simulink model "RL1"  (R2023a)
settings: Solver=FixedStepAuto  StartTime=0.0  StopTime=100  FixedStep=0.05  RelTol=1e-3  EnableMultiTasking=on
values from neighbouring files (symbols this model uses):
  Inz = 1538    [MAIN.m]
  Kx = zeros(n+1, n+1)    [MAIN.m]
  Kz = [K(2)      -K(2)    0         0         0         0    0 ... (first row only)    [MAIN.m]
  Mx = Mx + triu(Mx, 1)'    [MAIN.m]
  Mz = zeros(7,7)    [MAIN.m]
libraries: simulink x6, rllib x1
settings Model: ExtModeTrigDuration=10000  Creator=AUSIM-ZJD  LastModifiedBy=AUSIM-ZJD
settings SolverCC: AlgebraicLoopSolver=TrustRegion  PositivePriorityOrder=on
settings DataIOCC: ReturnWorkspaceOutputs=off
settings OptimizationCC: LifeSpan=inf
settings DebuggingCC: UnconnectedInputMsg=warning  UnconnectedOutputMsg=warning  UnconnectedLineMsg=warning  ArithmeticOperatorsInVariantConditions=warning
settings ModelReferenceCC: EnableRefExpFcnMdlSchedulingChecks=on
settings SFSimCC: SimUseLocalCustomCode=off  CustomCodeUndefinedFunction=UseInterfaceOnly
settings RTWCC: Description=QUARC Win64 Target  SystemTargetFile=quarc_win64.tlc  TemplateMakefile=quarc_default_tmf  RTWUseLocalCustomCode=off
settings CodeAppCC: StateflowObjectComments=on
settings STFCustomTargetCC: TargetPreCompLibLocation=C:\PROGRA~3\QUARC\lib\2016a\win64\release  UseToolchainInfoCompliant=off  SystemTargetFile=quarc_win64.tlc
settings GRTTargetCC: TargetPreCompLibLocation=C:\PROGRA~3\QUARC\lib\2016a\win64\release  ParMdlRefBuildCompliant=off  CompOptLevelCompliant=off  CombineOutputUpdateFcns=off  MatFileLogging=off  CPPClassGenCompliant=off  GRTInterface=on  UseToolchainInfoCompliant=off  ExtMode=on  ExtModeMexFile=quarc_comm
settings ConfigComp: CovMetricSettings=dswe

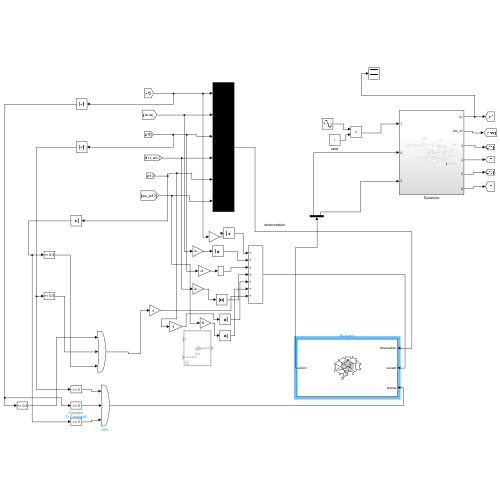
[thumbnail: Simulink's stored preview of the top-level diagram]
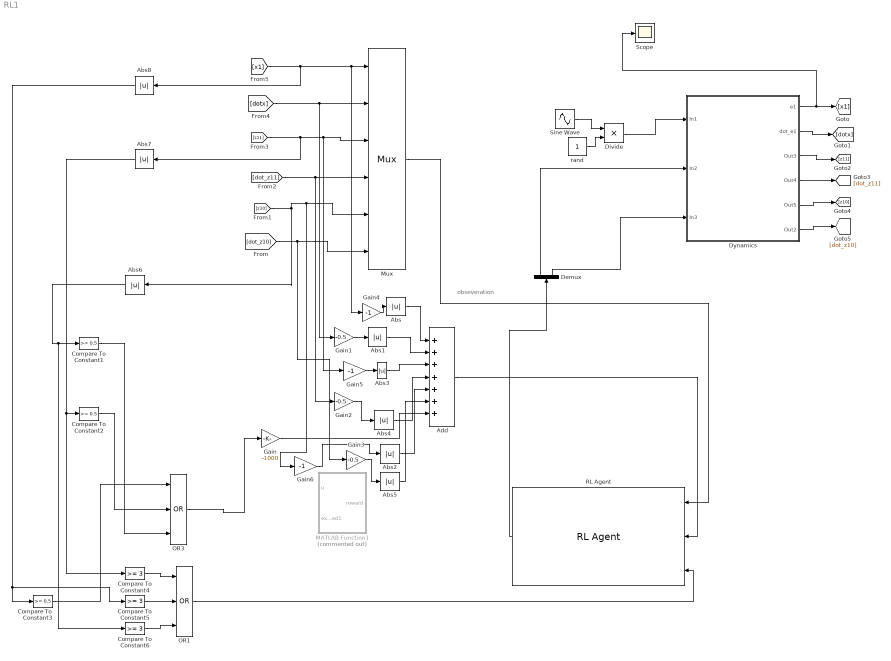
== system RL1 ==
  note: obseveration
  Abs{,1..8} (9 alike) : Abs  SaturateOnIntegerOverflow=off
  Add : Sum  Inputs=+++++++
  Compare To Constant1 : simulink/Logic and Bit Operations/Compare To Constant  relop=>=  const=0.5  OutDataTypeStr=boolean
  Compare To Constant2 : simulink/Logic and Bit Operations/Compare To Constant  relop=>=  const=0.5  OutDataTypeStr=boolean
  Compare To Constant3 : simulink/Logic and Bit Operations/Compare To Constant  relop=>=  const=0.5  OutDataTypeStr=boolean
  Compare To Constant4 : simulink/Logic and Bit Operations/Compare To Constant  relop=>=  const=3  OutDataTypeStr=boolean
  Compare To Constant5 : simulink/Logic and Bit Operations/Compare To Constant  relop=>=  const=3  OutDataTypeStr=boolean
  Compare To Constant6 : simulink/Logic and Bit Operations/Compare To Constant  relop=>=  const=3  OutDataTypeStr=boolean
  Demux : Demux  Outputs=2
  Divide : Product  Inputs=**
  Dynamics : Subsystem
  Gain : Gain  Gain=-1000
  Gain1 : Gain  Gain=-0.5
  Gain2 : Gain  Gain=-0.5
  Gain3 : Gain  Gain=-0.5
  Gain4 : Gain  Gain=-1
  Gain5 : Gain  Gain=-1
  Gain6 : Gain  Gain=-1
  MATLAB Function1 : MATLAB Function  Commented=on  TreatAsAtomicUnit=on
  Mux : Mux  Inputs=6
  OR1 : Logic  Operator=OR  Inputs=3  IconShape=distinctive  AllPortsSameDT=off  OutDataTypeStr=boolean
  OR3 : Logic  Operator=OR  Inputs=3  IconShape=distinctive  AllPortsSameDT=off  OutDataTypeStr=boolean
  RL Agent : rllib/RL Agent  Agent=agent  ExternalActionAsInput=off  ProvideLastAction=off  ProvideCumRwd=off  TreatAsDirectFeedthrough=on  UseStrictObservationDataTypes=off
  Scope : Scope
  Sine Wave : Sin  Amplitude=5000  SampleTime=0.05
  rand : Constant
  wires:
  Sine Wave/1 -> Divide/1
  Demux/2 -> Dynamics/3(In3)
  Dynamics/2(dot_e1) -> [dotx]
  Dynamics/6(Out2) -> [dot_z10]
  Dynamics/1(e1) -> Scope/1, [x1]
  Dynamics/3(Out3) -> [z11]
  Dynamics/4(Out4) -> [dot_z11]
  Dynamics/5(Out5) -> [z10]
  [dotx] -> Mux/2, Gain1/1
  [dot_z10] -> Gain3/1, Mux/6
  Mux/1 -> RL Agent/1
  [dot_z11] -> Gain2/1, Mux/4
  Add/1 -> RL Agent/2
  RL Agent/1 -> Demux/1
  Demux/1 -> Dynamics/2(In2)
  Compare To Constant1/1 -> OR3/3
  [z10] -> Gain6/1, Mux/5, Abs6/1
  Compare To Constant2/1 -> OR3/2
  [z11] -> Abs7/1, Gain5/1, Mux/3
  OR3/1 -> Gain/1
  Compare To Constant3/1 -> OR3/1
  [x1] -> Abs8/1, Mux/1, Gain4/1
  Divide/1 -> Dynamics/1(In1)
  rand/1 -> Divide/2
  Abs/1 -> Add/1
  Abs1/1 -> Add/2
  Abs3/1 -> Add/3
  Abs4/1 -> Add/4
  Abs2/1 -> Add/5
  Abs5/1 -> Add/6
  Gain/1 -> Add/7
  Abs6/1 -> Compare To Constant6/1, Compare To Constant1/1
  Abs7/1 -> Compare To Constant4/1, Compare To Constant2/1
  Abs8/1 -> Compare To Constant3/1, Compare To Constant5/1
  Gain1/1 -> Abs1/1
  Gain2/1 -> Abs4/1
  Gain3/1 -> Abs5/1
  Gain4/1 -> Abs/1
  Gain5/1 -> Abs3/1
  Gain6/1 -> Abs2/1
  Compare To Constant4/1 -> OR1/1
  Compare To Constant5/1 -> OR1/2
  Compare To Constant6/1 -> OR1/3
  OR1/1 -> RL Agent/3

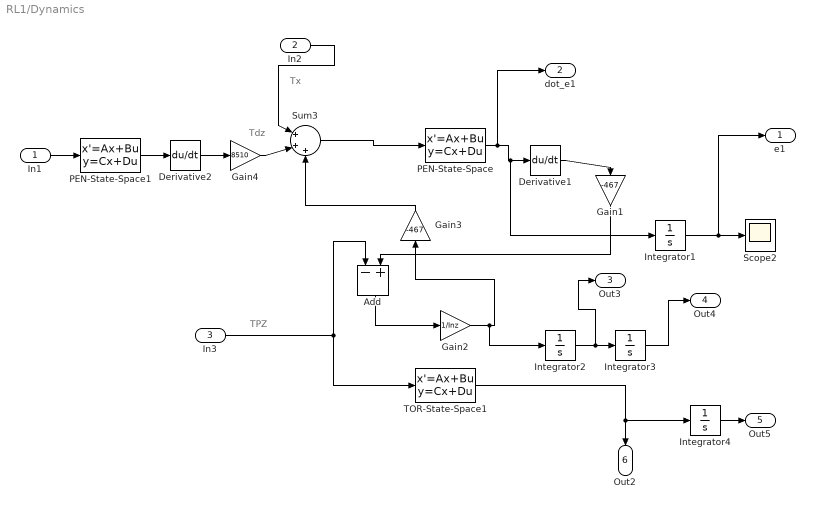
== system RL1/Dynamics ==
  note: TPZ
  note: Tx
  note: Tdz
  In1 : Inport
  In2 : Inport  Port=2
  In3 : Inport  Port=3
  Add : Sum  Inputs=-+
  Derivative1 : Derivative
  Derivative2 : Derivative
  Gain1 : Gain  Gain=-467
  Gain2 : Gain  Gain=1/Inz
  Gain3 : Gain  Gain=-467
  Gain4 : Gain  Gain=8510
  Integrator{1..4} (4 alike) : Integrator
  PEN-State-Space : StateSpace  A=[zeros(12, 12), eye(12); -Mx\Kx, zeros(12, 12)]  B=[zeros(12, 1); Mx\ [0; 0; 0; 0; 0; 0;0; 0; 0; 0; 0; 1]]  C=[ 0, 0, 0, 0, 0,0,0, 0, 0, 0, 0, 0, 0, 0, 0, 0, 0,0,0, 0, 0, 0, 0, 1]  D=0  InitialCondition=[0, 0, 0, 0, 0,0, 0,0, 0, 0, 0, 0, 0,0,0,0, 0,0, 0, 0, 0, 0, 0,0]
  PEN-State-Space1 : StateSpace  A=[zeros(12, 12), eye(12); -Mx\Kx, zeros(12, 12)]  B=[zeros(12, 1); Mx\ [1; 0; 0; 0; 0; 0;0; 0; 0; 0; 0; 0]]  C=[ 0, 0, 0, 0, 0,0,0, 0, 0, 0, 0, 0, 0, 0, 0, 0, 0,0,0, 0, 0, 0, 0, 1]  D=0  InitialCondition=[0, 0, 0, 0, 0,0, 0,0, 0, 0, 0, 0, 0,0,0,0, 0,0, 0, 0, 0, 0, 0,0]
  Scope2 : Scope
  Sum3 : Sum  Inputs=|+++
  TOR-State-Space1 : StateSpace  A=[zeros(7, 7), eye(7); -inv(Mz)*Kz, zeros(7, 7)]  B=[zeros(7, 1); inv(Mz) * [0; 0; 0; 0; 0; 0;1]]  C=[0, 0, 0, 0, 0, 0,0,0, 0, 0, 0, 0, 0, 1]  D=0  InitialCondition=[0, 0, 0, 0, 0,0, 0,0, 0, 0, 0, 0, 0,0]
  e1 : Outport
  dot_e1 : Outport  Port=2
  Out3 : Outport  Port=3
  Out4 : Outport  Port=4
  Out5 : Outport  Port=5
  Out2 : Outport  Port=6
  wires:
  In3/1 -> TOR-State-Space1/1, Add/1
  In1/1 -> PEN-State-Space1/1
  Gain1/1 -> Add/2
  Integrator1/1 -> e1/1, Scope2/1
  PEN-State-Space/1 -> dot_e1/1, Integrator1/1, Derivative1/1
  Gain2/1 -> Integrator2/1, Gain3/1
  In2/1 -> Sum3/1
  Derivative1/1 -> Gain1/1
  Add/1 -> Gain2/1
  Sum3/1 -> PEN-State-Space/1
  TOR-State-Space1/1 -> Integrator4/1, Out2/1
  Gain3/1 -> Sum3/3
  Integrator2/1 -> Out3/1, Integrator3/1
  Integrator3/1 -> Out4/1
  Integrator4/1 -> Out5/1
  PEN-State-Space1/1 -> Derivative2/1
  Derivative2/1 -> Gain4/1
  Gain4/1 -> Sum3/2

== matlab function RL1/MATLAB Function1 ==
  data: u input; reward output; exceed1 input
function reward = fcn(u,exceed1)
    
reward = -sum(abs(u(1))+abs(u(3))+abs(u(5)))-0.5*sum(abs(u(2))+abs(u(4))+abs(u(6)))-1000*abs(exceed1);
end
